simulink model "nmpc"  (R2021b)
settings: Solver=ode23s  StartTime=0.0  StopTime=120  FixedStep=0.0001  RelTol=1e-3
values from neighbouring files (symbols this model uses):
  Bf = 10000    [parameters.m]
  Bw = 1.7    [parameters.m]
  Hp = 23    [parameters.m]
  initial_speed = params(3)    [CustomCostFcn.m]    (also in parameters.m = 1.38888888889)
  initial_theta = deg2rad(9)    [parameters.m]
  initial_x = 0    [parameters.m]
  initial_y = 0.05    [parameters.m]
  J = sum((X(2:end,1) - data.References(:,1)).^2 + (X(2:end,2) - data.References(:,2)).^2 + (initial_speed*step_time*(X(2:end,3) - data.References(:,3))).^2 + ((initial_speed*step_time)^2/L*(X(2:end,4) - data.References(:,4))).^2)    [CustomCostFcn.m]    (also in parameters.m = 50)
  Jw = 5    [parameters.m]
  K = 1    [parameters.m]
  Kp = 20    [parameters.m]
  L = params(1)    [CarLikeRobot.m]    (also in CustomCostFcn.m; parameters.m = 1.58)
  Lf = 0.79    [parameters.m]
  Lr = 0.79    [parameters.m]
  Lw = 0.54    [parameters.m]
  M = 250    [parameters.m]
  omega_f = 0.3253    [parameters.m]
  phi_max = 0.61    [parameters.m]
  R = 0.29    [parameters.m]
  speed_allow_direction = 0.1407    [parameters.m]
  step_time = params(2)    [CustomCostFcn.m]    (also in parameters.m = 0.2)
  trajectory = trajectory_straight    [parameters.m]
undefined symbols (not defined in the file or in its folder): final_time
libraries: slpidlib x4, simulink x2, mpclib x1
settings Model: Creator=root  LastModifiedBy=roman
settings SolverCC: AlgebraicLoopSolver=TrustRegion
settings DataIOCC: ReturnWorkspaceOutputs=off  OutputOption=SpecifiedOutputTimes  OutputTimes=[0:0.01:(final_time*1.5)]
settings DebuggingCC: SFMachineParentedDataDiag=warning  ArithmeticOperatorsInVariantConditions=warning
settings SFSimCC: SimUseLocalCustomCode=off  CustomCodeUndefinedFunction=UseInterfaceOnly
settings RTWCC: RTWUseLocalCustomCode=off

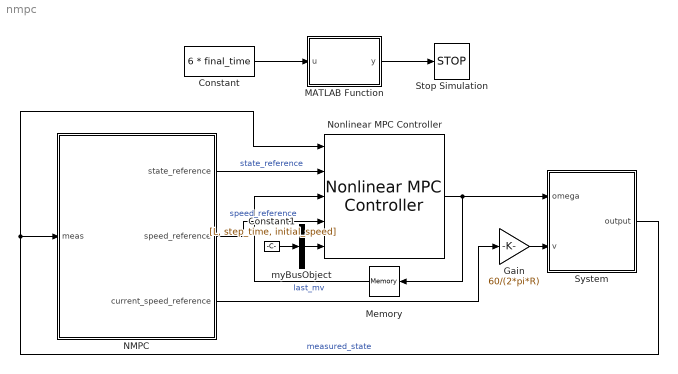
== system nmpc ==
  Constant : Constant  Value=6 * final_time
  Constant1 : Constant  Value=[L, step_time, initial_speed]
  Gain : Gain  Gain=60/(2*pi*R)
  MATLAB Function : MATLAB Function  TreatAsAtomicUnit=on
  Memory : Memory  InitialCondition=[0]
  NMPC : MATLAB Function  TreatAsAtomicUnit=on
  Nonlinear MPC Controller : mpclib/Nonlinear MPC Controller  nlmpcobj=nlobj  UseObjectTs=on  UseMEX=off  md_enabled=on  mvtarget_enabled=off  param_enabled=on  cost_enabled=off  mvseq_enabled=off  stateseq_enabled=off  ovseq_enabled=off  slack_enabled=off  status_enabled=off  ov_min=off  ov_max=off  mv_min=off  mv_max=off  mvrate_min=off  mvrate_max=off  state_min=off  state_max=off  ov_weight=off  mv_weight=off  mvrate_weight=off  ecr_weight=off  nlp_initialize=off
  Stop Simulation : Stop
  System : Subsystem
  myBusObject : BusCreator  Inputs=1  OutDataTypeStr=Bus: myBusObject  NonVirtualBus=on
      settings: InheritFromInputs=off
  wires:
  System/1(output) -> Nonlinear MPC Controller/1, NMPC/1(meas)  "measured_state"
  Memory/1 -> Nonlinear MPC Controller/3  "last_mv"
  NMPC/1(state_reference) -> Nonlinear MPC Controller/2  "state_reference"
  Nonlinear MPC Controller/1 -> System/1(omega), Memory/1
  NMPC/2(speed_reference) -> Nonlinear MPC Controller/4  "speed_reference"
  NMPC/3(current_speed_reference) -> Gain/1
  Gain/1 -> System/2(v)
  MATLAB Function/1(y) -> Stop Simulation/1
  Constant/1 -> MATLAB Function/1(u)
  myBusObject/1 -> Nonlinear MPC Controller/5
  Constant1/1 -> myBusObject/1

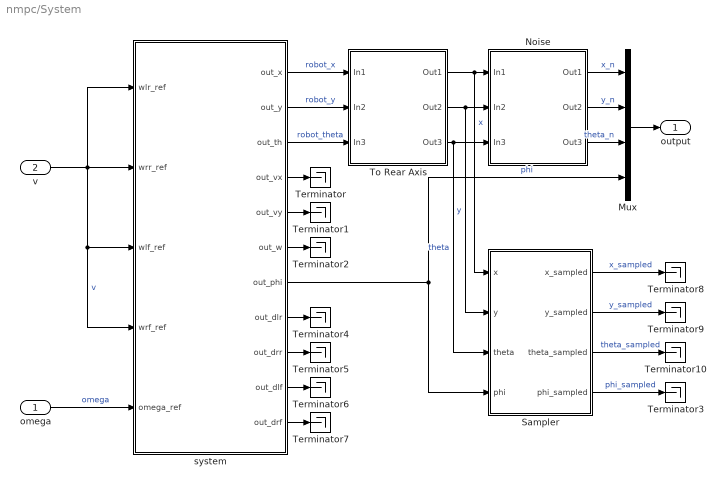
== system nmpc/System ==
  omega : Inport
  v : Inport  Port=2
  Mux : Mux
  Noise : Subsystem
  Sampler : MATLAB Function  TreatAsAtomicUnit=on
  Terminator{,1..10} (11 alike) : Terminator
  To Rear Axis : Subsystem
  system : Subsystem
  output : Outport  VectorParamsAs1DForOutWhenUnconnected=off
  wires:
  v/1 -> system/4(wrf_ref), system/3(wlf_ref), system/2(wrr_ref), system/1(wlr_ref)  "v"
  system/1(out_x) -> To Rear Axis/1(In1)  "robot_x"
  system/2(out_y) -> To Rear Axis/2(In2)  "robot_y"
  system/3(out_th) -> To Rear Axis/3(In3)  "robot_theta"
  omega/1 -> system/5(omega_ref)  "omega"
  Mux/1 -> output/1
  Noise/1(Out1) -> Mux/1  "x_n"
  Noise/2(Out2) -> Mux/2  "y_n"
  Noise/3(Out3) -> Mux/3  "theta_n"
  system/4(out_vx) -> Terminator/1
  system/5(out_vy) -> Terminator1/1
  system/6(out_w) -> Terminator2/1
  system/8(out_dlr) -> Terminator4/1
  system/9(out_drr) -> Terminator5/1
  system/10(out_dlf) -> Terminator6/1
  system/11(out_drf) -> Terminator7/1
  To Rear Axis/3(Out3) -> Noise/3(In3), Sampler/3(theta)  "theta"
  To Rear Axis/2(Out2) -> Noise/2(In2), Sampler/2(y)  "y"
  To Rear Axis/1(Out1) -> Noise/1(In1), Sampler/1(x)  "x"
  Sampler/1(x_sampled) -> Terminator8/1  "x_sampled"
  Sampler/2(y_sampled) -> Terminator9/1  "y_sampled"
  Sampler/3(theta_sampled) -> Terminator10/1  "theta_sampled"
  system/7(out_phi) -> Mux/4, Sampler/4(phi)  "phi"
  Sampler/4(phi_sampled) -> Terminator3/1  "phi_sampled"

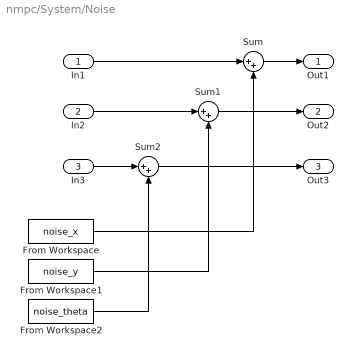
== system nmpc/System/Noise ==
  In1 : Inport
  In2 : Inport  Port=2
  In3 : Inport  Port=3
  From Workspace : FromWorkspace  VariableName=noise_x  SampleTime=step_time  OutputAfterFinalValue=Holding final value
  From Workspace1 : FromWorkspace  VariableName=noise_y  SampleTime=step_time  OutputAfterFinalValue=Holding final value
  From Workspace2 : FromWorkspace  VariableName=noise_theta  SampleTime=step_time  OutputAfterFinalValue=Holding final value
  Sum : Sum  Inputs=|++
  Sum1 : Sum  Inputs=|++
  Sum2 : Sum  Inputs=|++
  Out1 : Outport  VectorParamsAs1DForOutWhenUnconnected=off
  Out2 : Outport  Port=2  VectorParamsAs1DForOutWhenUnconnected=off
  Out3 : Outport  Port=3  VectorParamsAs1DForOutWhenUnconnected=off
  wires:
  Sum1/1 -> Out2/1
  In2/1 -> Sum1/1
  Sum/1 -> Out1/1
  In3/1 -> Sum2/1
  From Workspace/1 -> Sum/2
  From Workspace1/1 -> Sum1/2
  In1/1 -> Sum/1
  From Workspace2/1 -> Sum2/2
  Sum2/1 -> Out3/1

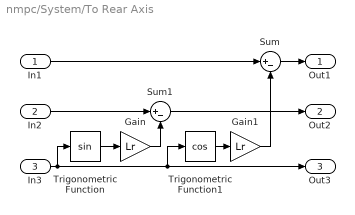
== system nmpc/System/To Rear Axis ==
  In1 : Inport
  In2 : Inport  Port=2
  In3 : Inport  Port=3
  Gain : Gain  Gain=Lr
  Gain1 : Gain  Gain=Lr
  Sum : Sum  Inputs=|+-
  Sum1 : Sum  Inputs=|+-
  Trigonometric Function : Trigonometry
  Trigonometric Function1 : Trigonometry  Operator=cos
  Out1 : Outport  VectorParamsAs1DForOutWhenUnconnected=off
  Out2 : Outport  Port=2  VectorParamsAs1DForOutWhenUnconnected=off
  Out3 : Outport  Port=3  VectorParamsAs1DForOutWhenUnconnected=off
  wires:
  In1/1 -> Sum/1
  In2/1 -> Sum1/1
  Sum/1 -> Out1/1
  Sum1/1 -> Out2/1
  Trigonometric Function/1 -> Gain/1
  Gain/1 -> Sum1/2
  In3/1 -> Out3/1, Trigonometric Function1/1, Trigonometric Function/1
  Trigonometric Function1/1 -> Gain1/1
  Gain1/1 -> Sum/2

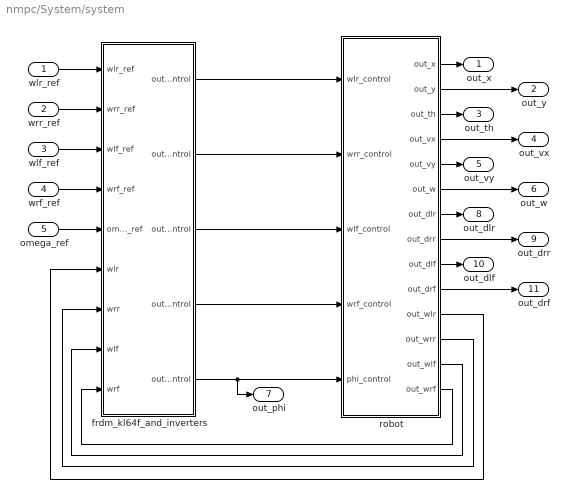
== system nmpc/System/system ==
  wlr_ref : Inport
  wrr_ref : Inport  Port=2
  wlf_ref : Inport  Port=3
  wrf_ref : Inport  Port=4
  omega_ref : Inport  Port=5
  frdm_kl64f_and_inverters : Subsystem
  robot : Subsystem
  out_x : Outport  VectorParamsAs1DForOutWhenUnconnected=off
  out_y : Outport  Port=2  VectorParamsAs1DForOutWhenUnconnected=off
  out_th : Outport  Port=3  VectorParamsAs1DForOutWhenUnconnected=off
  out_vx : Outport  Port=4  VectorParamsAs1DForOutWhenUnconnected=off
  out_vy : Outport  Port=5  VectorParamsAs1DForOutWhenUnconnected=off
  out_w : Outport  Port=6  VectorParamsAs1DForOutWhenUnconnected=off
  out_phi : Outport  Port=7  VectorParamsAs1DForOutWhenUnconnected=off
  out_dlr : Outport  Port=8  VectorParamsAs1DForOutWhenUnconnected=off
  out_drr : Outport  Port=9  VectorParamsAs1DForOutWhenUnconnected=off
  out_dlf : Outport  Port=10  VectorParamsAs1DForOutWhenUnconnected=off
  out_drf : Outport  Port=11  VectorParamsAs1DForOutWhenUnconnected=off
  wires:
  wlr_ref/1 -> frdm_kl64f_and_inverters/1(wlr_ref)
  wrr_ref/1 -> frdm_kl64f_and_inverters/2(wrr_ref)
  wlf_ref/1 -> frdm_kl64f_and_inverters/3(wlf_ref)
  wrf_ref/1 -> frdm_kl64f_and_inverters/4(wrf_ref)
  omega_ref/1 -> frdm_kl64f_and_inverters/5(omega_ref)
  robot/11(out_wlr) -> frdm_kl64f_and_inverters/6(wlr)
  robot/12(out_wrr) -> frdm_kl64f_and_inverters/7(wrr)
  robot/13(out_wlf) -> frdm_kl64f_and_inverters/8(wlf)
  robot/14(out_wrf) -> frdm_kl64f_and_inverters/9(wrf)
  frdm_kl64f_and_inverters/1(outwlr_control) -> robot/1(wlr_control)
  frdm_kl64f_and_inverters/2(outwrr_control) -> robot/2(wrr_control)
  frdm_kl64f_and_inverters/3(outwlf_control) -> robot/3(wlf_control)
  frdm_kl64f_and_inverters/4(outwrf_control) -> robot/4(wrf_control)
  robot/1(out_x) -> out_x/1
  robot/2(out_y) -> out_y/1
  robot/3(out_th) -> out_th/1
  robot/5(out_vy) -> out_vy/1
  robot/7(out_dlr) -> out_dlr/1
  robot/9(out_dlf) -> out_dlf/1
  robot/10(out_drf) -> out_drf/1
  robot/8(out_drr) -> out_drr/1
  robot/6(out_w) -> out_w/1
  robot/4(out_vx) -> out_vx/1
  frdm_kl64f_and_inverters/5("outphi_control ") -> robot/5(phi_control), out_phi/1

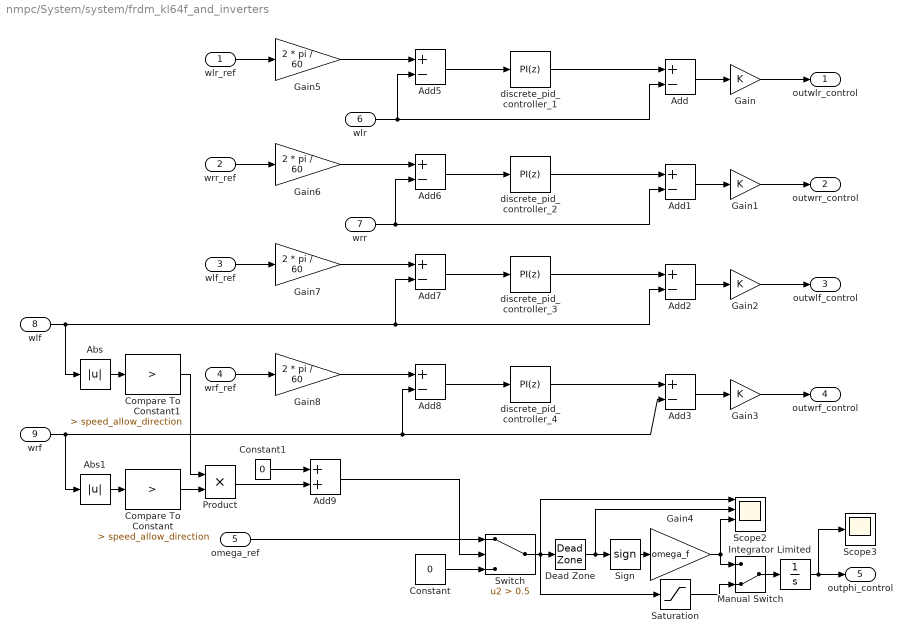
== system nmpc/System/system/frdm_kl64f_and_inverters ==
  wlr_ref : Inport
  wrr_ref : Inport  Port=2
  wlf_ref : Inport  Port=3
  wrf_ref : Inport  Port=4
  omega_ref : Inport  Port=5
  wlr : Inport  Port=6
  wrr : Inport  Port=7
  wlf : Inport  Port=8
  wrf : Inport  Port=9
  Abs : Abs
  Abs1 : Abs
  Add{,1..3,5..8} (8 alike) : Sum  Inputs=+-
  Add9 : Sum
  Compare To Constant : simulink/Logic and Bit Operations/Compare To Constant  relop=>  const=speed_allow_direction  OutDataTypeStr=boolean
  Compare To Constant1 : simulink/Logic and Bit Operations/Compare To Constant  relop=>  const=speed_allow_direction  OutDataTypeStr=boolean
  Constant : Constant  Value=0
  Constant1 : Constant  Value=0
  Dead Zone : DeadZone  LowerValue=-omega_f/2  UpperValue=omega_f/2  SaturateOnIntegerOverflow=on
  Gain{,1..3} (4 alike) : Gain  Gain=K
  Gain4 : Gain  Gain=omega_f
  Gain{5..8} (4 alike) : Gain  Gain=2 * pi / 60
  Integrator Limited : Integrator  LimitOutput=on  UpperSaturationLimit=phi_max  LowerSaturationLimit=-phi_max
  Manual Switch : ManualSwitch  CurrentSetting=0
  Product : Product
  Saturation : Saturate  UpperLimit=omega_f  LowerLimit=-omega_f
  Scope2 : Scope  NumInputPorts=4
  Scope3 : Scope
  Sign : Signum
  Switch : Switch  Criteria=u2 > Threshold  Threshold=0.5
  discrete_pid_controller_{1..4} (4 alike) : slpidlib/PID Controller  Controller=PI  Form=Parallel  TimeDomain=Discrete-time  UseExternalTs=off  SampleTime=step_time  IntegratorMethod=Forward Euler  FilterMethod=Forward Euler  ControllerParametersSource=internal  P=Kp  I=Kp / Ti  D=0  UseFilter=off  N=100  TunerSelectOption=Transfer Function Based (PID Tuner App)  InitialConditionSource=internal  InitialConditionForIntegrator=0  InitialConditionForFilter=0  DifferentiatorICPrevScaledInput=0  ExternalReset=none  TrackingMode=off  Kt=1  LimitOutput=off  SatLimitsSource=internal  UpperSaturationLimit=inf  LowerSaturationLimit=-inf  LinearizeAsGain=off  AntiWindupMode=none  Kb=1  POutMin=[]  POutMax=[]  IOutMin=[]  IOutMax=[]  DOutMin=[]  DOutMax=[]  NOutMin=[]  NOutMax=[]  SumOutMin=[]  SumOutMax=[]  SaturationOutMin=[]  SaturationOutMax=[]  PParamMin=[]  PParamMax=[]  IParamMin=[]  IParamMax=[]  DParamMin=[]  DParamMax=[]  NParamMin=[]  NParamMax=[]  KbParamMin=[]  KbParamMax=[]  KtParamMin=[]  KtParamMax=[]  KbOutMin=[]  KbOutMax=[]  KtOutMin=[]  KtOutMax=[]  IntegratorOutMin=[]  IntegratorOutMax=[]  FilterOutMin=[]  FilterOutMax=[]  SumI1OutMin=[]  SumI1OutMax=[]  SumI2OutMin=[]  SumI2OutMax=[]  SumI3OutMin=[]  SumI3OutMax=[]  SumI4OutMin=[]  SumI4OutMax=[]  SumDOutMin=[]  SumDOutMax=[]  DifferentiatorOutMin=[]  DifferentiatorOutMax=[]  FilterDiffOutCoefMin=[]  FilterDiffOutCoefMax=[]  ReciprocalOutMin=[]  ReciprocalOutMax=[]  SumDenOutMin=[]  SumDenOutMax=[]  SumNumOutMin=[]  SumNumOutMax=[]  DivideOutMin=[]  DivideOutMax=[]  UdiffTsProdOutMin=[]  UdiffTsProdOutMax=[]  NTsProdOutMin=[]  NTsProdOutMax=[]  UintegralTsProdOutMin=[]  UintegralTsProdOutMax=[]  UngainTsProdOutMin=[]  UngainTsProdOutMax=[]  IntegratorContinuousStateAttributes=''  IntegratorStateMustResolveToSignalObject=off  IntegratorRTWStateStorageClass=Auto  FilterContinuousStateAttributes=''  FilterStateMustResolveToSignalObject=off  FilterRTWStateStorageClass=Auto  ParallelPVariant=InternalParameters  IdealPVariant=Disabled  IVariant=InternalParameters  DVariant=Disabled  IntegratorVariant=Discrete  SatVariant=Disabled  AWVariant=Passthrough  PCopyVariant=Disabled  TRVariant=Disabled  FdbkBlocksVariant=Forward  IdealPFdbkVariant=Disabled  SatFdbkVariant=Disabled  DerivativeFilterVariant=Disabled  NVariant=Disabled  NCopyVariant=Disabled_SignalSpec  FilterICVariant=Disabled  IntegratorICVariant=InternalICs  ExternalResetVariant=Disabled  TRSumVariant=Passthrough  SumFdbkVariant=Disabled  SumVariant=Sum_PI  TsampFilterVariant=InternalTs  TsampNgainVariant=Passthrough  TsampIntegralVariant=Passthrough  ExternalSaturationOutDataTypeStr=Inherit: Same as second input
  outwlr_control : Outport  VectorParamsAs1DForOutWhenUnconnected=off
  outwrr_control : Outport  Port=2  VectorParamsAs1DForOutWhenUnconnected=off
  outwlf_control : Outport  Port=3  VectorParamsAs1DForOutWhenUnconnected=off
  outwrf_control : Outport  Port=4  VectorParamsAs1DForOutWhenUnconnected=off
  "outphi_control " : Outport  Port=5  VectorParamsAs1DForOutWhenUnconnected=off
  wires:
  Gain2/1 -> outwlf_control/1
  Gain4/1 -> Scope2/3, Manual Switch/1
  wrf/1 -> Abs1/1, Add8/2, Add3/2
  Sign/1 -> Gain4/1
  wrr/1 -> Add6/2, Add1/2
  Add7/1 -> discrete_pid_controller_3/1
  Add6/1 -> discrete_pid_controller_2/1
  Add3/1 -> Gain3/1
  wlr/1 -> Add5/2, Add/2
  Add/1 -> Gain/1
  Add1/1 -> Gain1/1
  wlf/1 -> Abs/1, Add7/2, Add2/2
  Add5/1 -> discrete_pid_controller_1/1
  discrete_pid_controller_4/1 -> Add3/1
  Add2/1 -> Gain2/1
  discrete_pid_controller_2/1 -> Add1/1
  Gain/1 -> outwlr_control/1
  Integrator Limited/1 -> Scope3/1, "outphi_control "/1
  discrete_pid_controller_3/1 -> Add2/1
  Add8/1 -> discrete_pid_controller_4/1
  Gain3/1 -> outwrf_control/1
  discrete_pid_controller_1/1 -> Add/1
  Gain1/1 -> outwrr_control/1
  wlr_ref/1 -> Gain5/1
  Gain5/1 -> Add5/1
  wrr_ref/1 -> Gain6/1
  Gain6/1 -> Add6/1
  wlf_ref/1 -> Gain7/1
  Gain7/1 -> Add7/1
  wrf_ref/1 -> Gain8/1
  Gain8/1 -> Add8/1
  Compare To Constant/1 -> Product/2
  Compare To Constant1/1 -> Product/1
  omega_ref/1 -> Switch/1
  Constant/1 -> Switch/3
  Abs/1 -> Compare To Constant1/1
  Abs1/1 -> Compare To Constant/1
  Dead Zone/1 -> Sign/1, Scope2/2
  Add9/1 -> Switch/2
  Constant1/1 -> Add9/1
  Product/1 -> Add9/2
  Manual Switch/1 -> Integrator Limited/1
  Switch/1 -> Saturation/1, Dead Zone/1, Scope2/1
  Saturation/1 -> Manual Switch/2

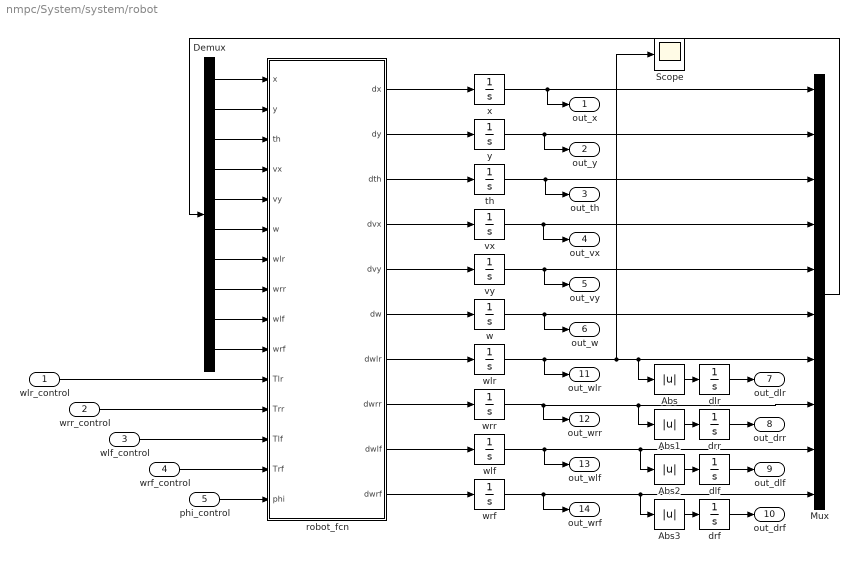
== system nmpc/System/system/robot ==
  wlr_control : Inport
  wrr_control : Inport  Port=2
  wlf_control : Inport  Port=3
  wrf_control : Inport  Port=4
  phi_control : Inport  Port=5
  Abs{,1..3} (4 alike) : Abs
  Demux : Demux  Outputs=10
  Mux : Mux  Inputs=10
  Scope : Scope
  dlf : Integrator
  dlr : Integrator
  drf : Integrator
  drr : Integrator
  robot_fcn : MATLAB Function  TreatAsAtomicUnit=on
  th : Integrator  InitialCondition=initial_theta
  vx : Integrator
  vy : Integrator
  w : Integrator
  wlf : Integrator
  wlr : Integrator
  wrf : Integrator
  wrr : Integrator
  x : Integrator  InitialCondition=initial_x + Lr * cos(initial_theta)
  y : Integrator  InitialCondition=initial_y + Lr * sin(initial_theta)
  out_x : Outport  VectorParamsAs1DForOutWhenUnconnected=off
  out_y : Outport  Port=2  VectorParamsAs1DForOutWhenUnconnected=off
  out_th : Outport  Port=3  VectorParamsAs1DForOutWhenUnconnected=off
  out_vx : Outport  Port=4  VectorParamsAs1DForOutWhenUnconnected=off
  out_vy : Outport  Port=5  VectorParamsAs1DForOutWhenUnconnected=off
  out_w : Outport  Port=6  VectorParamsAs1DForOutWhenUnconnected=off
  out_dlr : Outport  Port=7  VectorParamsAs1DForOutWhenUnconnected=off
  out_drr : Outport  Port=8  VectorParamsAs1DForOutWhenUnconnected=off
  out_dlf : Outport  Port=9  VectorParamsAs1DForOutWhenUnconnected=off
  out_drf : Outport  Port=10  VectorParamsAs1DForOutWhenUnconnected=off
  out_wlr : Outport  Port=11  VectorParamsAs1DForOutWhenUnconnected=off
  out_wrr : Outport  Port=12  VectorParamsAs1DForOutWhenUnconnected=off
  out_wlf : Outport  Port=13  VectorParamsAs1DForOutWhenUnconnected=off
  out_wrf : Outport  Port=14  VectorParamsAs1DForOutWhenUnconnected=off
  wires:
  robot_fcn/1(dx) -> x/1
  drr/1 -> out_drr/1
  dlf/1 -> out_dlf/1
  Demux/8 -> robot_fcn/8(wrr)
  robot_fcn/6(dw) -> w/1
  th/1 -> out_th/1, Mux/3
  w/1 -> out_w/1, Mux/6
  wlf/1 -> out_wlf/1, Abs2/1, Mux/9
  y/1 -> out_y/1, Mux/2
  Mux/1 -> Demux/1
  robot_fcn/10(dwrf) -> wrf/1
  vy/1 -> Mux/5, out_vy/1
  vx/1 -> Mux/4, out_vx/1
  Demux/1 -> robot_fcn/1(x)
  robot_fcn/9(dwlf) -> wlf/1
  drf/1 -> out_drf/1
  Demux/5 -> robot_fcn/5(vy)
  robot_fcn/2(dy) -> y/1
  Demux/2 -> robot_fcn/2(y)
  robot_fcn/8(dwrr) -> wrr/1
  wrr_control/1 -> robot_fcn/12(Trr)
  wrf_control/1 -> robot_fcn/14(Trf)
  phi_control/1 -> robot_fcn/15(phi)
  Demux/9 -> robot_fcn/9(wlf)
  x/1 -> out_x/1, Mux/1
  robot_fcn/7(dwlr) -> wlr/1
  robot_fcn/5(dvy) -> vy/1
  Demux/6 -> robot_fcn/6(w)
  robot_fcn/4(dvx) -> vx/1
  Demux/10 -> robot_fcn/10(wrf)
  robot_fcn/3(dth) -> th/1
  wlf_control/1 -> robot_fcn/13(Tlf)
  Demux/7 -> robot_fcn/7(wlr)
  Demux/4 -> robot_fcn/4(vx)
  wrf/1 -> out_wrf/1, Abs3/1, Mux/10
  Demux/3 -> robot_fcn/3(th)
  wrr/1 -> out_wrr/1, Abs1/1, Mux/8
  dlr/1 -> out_dlr/1
  wlr_control/1 -> robot_fcn/11(Tlr)
  Abs/1 -> dlr/1
  Abs1/1 -> drr/1
  Abs2/1 -> dlf/1
  Abs3/1 -> drf/1
  wlr/1 -> out_wlr/1, Scope/1, Abs/1, Mux/7

== matlab function nmpc/System/Sampler ==
  settings: updateMethod=DISCRETE  sampleTime=step_time/sampling_scale
  data: x input; y input; theta input; x_sampled output; y_sampled output; theta_sampled output; phi input; phi_sampled output
function [x_sampled,y_sampled, theta_sampled, phi_sampled] = fcn(x, y, theta, phi)
x_sampled = x;
y_sampled = y;
theta_sampled = theta;
phi_sampled = phi;

== matlab function nmpc/NMPC ==
  settings: updateMethod=DISCRETE  sampleTime=step_time
  data: meas input; trajectory parameter; Hp parameter; step_time parameter; L parameter; state_reference output; speed_reference output; current_speed_reference output
function [state_reference, speed_reference, current_speed_reference] = fcn(meas, trajectory, Hp, step_time, L)
    coder.extrinsic('NmpcController');
    p = Hp;
    state_reference = zeros(p,4);
    speed_reference = zeros(p,1);
    current_speed_reference = 0;
    [state_reference, speed_reference, current_speed_reference] = NmpcController(meas, trajectory, Hp, step_time, L);

== matlab function nmpc/MATLAB Function ==
  data: u input; y output
function y = fcn(u)
    persistent first_time;
    if isempty(first_time)
        tic;
        first_time = 1;
    end
    y = toc > u;

== matlab function nmpc/System/system/robot/robot_fcn ==
  data: x input; dx output; y input; th input; vx input; vy input; w input; wlr input; wrr input; wlf input; wrf input; Tlr input; Trr input; Tlf input; Trf input; phi input; dy output; dth output; dvx output; dvy output; dw output; dwlr output; dwrr output; dwlf output; dwrf output; Lr parameter; Lf parameter; Lw parameter; R parameter; M parameter; J parameter; Jw parameter; Bw parameter; Bf parameter
function [dx, dy, dth, dvx, dvy, dw, dwlr, dwrr, dwlf, dwrf] = fcn(x, y, th, vx, vy, w, wlr, wrr, wlf, wrf, Tlr, Trr, Tlf, Trf, phi, Lr, Lf, Lw, R, M, J, Jw, Bw, Bf)
  
vxlr = vx + (Lr * sin(th) - Lw * cos(th)) * w;
vxrr = vx + (Lr * sin(th) + Lw * cos(th)) * w;
vxlf = vx + (-Lf * sin(th) - Lw * cos(th)) * w;
vxrf = vx + (-Lf * sin(th) + Lw * cos(th)) * w;
vylr = vy + (-Lr * cos(th) - Lw * sin(th)) * w;
vyrr = vy + (-Lr * cos(th) + Lw * sin(th)) * w;
vylf = vy + (Lf * cos(th) - Lw * sin(th)) * w;
vyrf = vy + (Lf * cos(th) + Lw * sin(th)) * w;

Fxlr = Bf * (R * wlr * cos(th) - vxlr);
Fylr = Bf * (R * wlr * sin(th) - vylr);
Fxrr = Bf * (R * wrr * cos(th) - vxrr);
Fyrr = Bf * (R * wrr * sin(th) - vyrr);
Fxlf = Bf * (R * wlf * cos(th + phi) - vxlf);
Fylf = Bf * (R * wlf * sin(th + phi) - vylf);
Fxrf = Bf * (R * wrf * cos(th + phi) - vxrf);
Fyrf = Bf * (R * wrf * sin(th + phi) - vyrf);

taulr = Fxlr * sin(th) * Lr - Fxlr * cos(th) * Lw - Fylr * cos(th) * Lr - Fylr * sin(th) * Lw;
taurr = Fxrr * sin(th) * Lr + Fxrr * cos(th) * Lw - Fyrr * cos(th) * Lr + Fyrr * sin(th) * Lw;
taulf = -Fxlf * sin(th) * Lf - Fxlf * cos(th) * Lw + Fylf * cos(th) * Lf - Fylf * sin(th) * Lw;
taurf = -Fxrf * sin(th) * Lf + Fxrf * cos(th) * Lw + Fyrf * cos(th) * Lf + Fylf * sin(th) * Lw;

dx = vx;
dy = vy;
dth = w;
dvx = (Fxlr + Fxrr + Fxlf + Fxrf) / M;
dvy = (Fylr + Fyrr + Fylf + Fyrf) / M;
dw = (taulr + taurr + taulf + taurf) / J;

dwlr = (Tlr - R * Fxlr * cos(th) - R * Fylr * sin(th) - Bw * wlr) / Jw;
dwrr = (Trr - R * Fxrr * cos(th) - R * Fyrr * sin(th) - Bw * wrr) / Jw;
dwlf = (Tlf - R * Fxlf * cos(th + phi) - R * Fylf * sin(th + phi) - Bw * wlf) / Jw;
dwrf = (Trf - R * Fxrf * cos(th + phi) - R * Fyrf * sin(th + phi) - Bw * wrf) / Jw;
